simulink model "mamapwm"  (R2013a)
settings: Solver=ode45  StartTime=0.0  StopTime=1.4  RelTol=1e-3
libraries: simulink x1
settings Model: Creator=leGaly  LastModifiedBy=leGaly

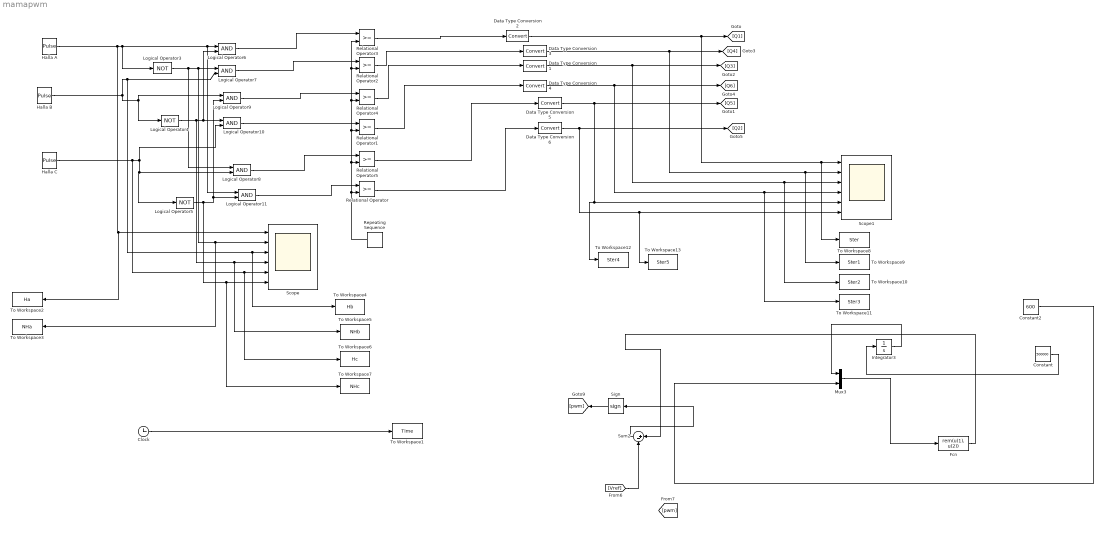
== system mamapwm ==
  Clock : Clock
  Constant : Constant  Value=500000
  Constant2 : Constant  Value=600
  Data Type Conversion{1..6} (6 alike) : DataTypeConversion
  Fcn : Fcn  Expr=rem(u(1), u(2))
  Halla A : DiscretePulseGenerator  PulseType=Time based  Period=0.6  PulseWidth=50
  Halla B : DiscretePulseGenerator  PulseType=Time based  Period=0.6  PulseWidth=50  PhaseDelay=0.2
  Halla C : DiscretePulseGenerator  PulseType=Time based  Period=0.6  PulseWidth=50  PhaseDelay=-0.2
  Integrator3 : Integrator
  Logical Operator{6..11} (6 alike) : Logic  AllPortsSameDT=off  OutDataTypeStr=boolean
  Logical Operator3 : Logic  Operator=NOT  AllPortsSameDT=off  OutDataTypeStr=boolean
  Logical Operator4 : Logic  Operator=NOT  AllPortsSameDT=off  OutDataTypeStr=boolean
  Logical Operator5 : Logic  Operator=NOT  AllPortsSameDT=off  OutDataTypeStr=boolean
  Mux3 : Mux  Inputs=2
  Relational Operator{,1..5} (6 alike) : RelationalOperator  OutDataTypeStr=boolean
  Repeating Sequence : simulink/Sources/Repeating Sequence  rep_seq_t=[0 12e-12]  rep_seq_y=[0.0001 1.5]
  Scope : Scope  NumInputPorts=6
      settings: YMin=-5~-5~-5~-5~-5~-5  YMax=5~5~5~5~5~5
  Scope1 : Scope  NumInputPorts=6
      settings: YMin=-5~-5~-5~-5~-5~-5  YMax=5~5~5~5~5~5
  Sign : Signum
  Sum2 : Sum  Inputs=|+-
  To Workspace1 : ToWorkspace  VariableName=Time  SampleTime=-1  SaveFormat=Structure With Time
  To Workspace10 : ToWorkspace  VariableName=Ster2  SampleTime=-1  SaveFormat=Structure With Time
  To Workspace11 : ToWorkspace  VariableName=Ster3  SampleTime=-1  SaveFormat=Structure With Time
  To Workspace12 : ToWorkspace  VariableName=Ster4  SampleTime=-1  SaveFormat=Structure With Time
  To Workspace13 : ToWorkspace  VariableName=Ster5  SampleTime=-1  SaveFormat=Structure With Time
  To Workspace2 : ToWorkspace  VariableName=Ha  SampleTime=-1  SaveFormat=Structure With Time
  To Workspace3 : ToWorkspace  VariableName=NHa  SampleTime=-1  SaveFormat=Structure With Time
  To Workspace4 : ToWorkspace  VariableName=Hb  SampleTime=-1  SaveFormat=Structure With Time
  To Workspace5 : ToWorkspace  VariableName=NHb  SampleTime=-1  SaveFormat=Structure With Time
  To Workspace6 : ToWorkspace  VariableName=Hc  SampleTime=-1  SaveFormat=Structure With Time
  To Workspace7 : ToWorkspace  VariableName=NHc  SampleTime=-1  SaveFormat=Structure With Time
  To Workspace8 : ToWorkspace  VariableName=Ster  SampleTime=-1  SaveFormat=Structure With Time
  To Workspace9 : ToWorkspace  VariableName=Ster1  SampleTime=-1  SaveFormat=Structure With Time
  wires:
  Logical Operator4/1 -> To Workspace5/1, Scope/4, Logical Operator10/1, Logical Operator6/2
  Logical Operator3/1 -> To Workspace3/1, Scope/2, Logical Operator7/1, Logical Operator8/1
  Logical Operator5/1 -> To Workspace7/1, Scope/6, Logical Operator11/2, Logical Operator9/2
  Logical Operator6/1 -> Relational Operator3/1
  Logical Operator9/1 -> Relational Operator4/1
  Logical Operator10/1 -> Relational Operator1/1
  Logical Operator8/1 -> Relational Operator5/1
  Logical Operator11/1 -> Relational Operator/1
  Halla A/1 -> To Workspace2/1, Scope/1, Logical Operator3/1, Logical Operator11/1, Logical Operator6/1
  Halla B/1 -> To Workspace4/1, Scope/3, Logical Operator7/2, Logical Operator4/1, Logical Operator9/1
  Halla C/1 -> To Workspace6/1, Scope/5, Logical Operator5/1, Logical Operator8/2, Logical Operator10/2
  Constant/1 -> Integrator3/1
  Integrator3/1 -> Mux3/1
  Constant2/1 -> Mux3/2
  Mux3/1 -> Fcn/1
  Fcn/1 -> Sum2/1
  Sum2/1 -> Sign/1
  Sign/1 -> [pwm]
  [Vref] -> Sum2/2
  Data Type Conversion2/1 -> To Workspace8/1, Scope1/1, [Q1]
  Data Type Conversion3/1 -> To Workspace9/1, Scope1/2, [Q4]
  Data Type Conversion1/1 -> To Workspace10/1, Scope1/3, [Q3]
  Data Type Conversion4/1 -> To Workspace11/1, Scope1/4, [Q6]
  Data Type Conversion5/1 -> Scope1/5, To Workspace12/1, [Q5]
  Data Type Conversion6/1 -> To Workspace13/1, Scope1/6, [Q2]
  Clock/1 -> To Workspace1/1
  Logical Operator7/1 -> Relational Operator2/1
  Relational Operator2/1 -> Data Type Conversion3/1
  Relational Operator3/1 -> Data Type Conversion2/1
  Repeating Sequence/1 -> Relational Operator/2, Relational Operator5/2, Relational Operator1/2, Relational Operator4/2, Relational Operator2/2, Relational Operator3/2
  Relational Operator4/1 -> Data Type Conversion1/1
  Relational Operator1/1 -> Data Type Conversion4/1
  Relational Operator5/1 -> Data Type Conversion5/1
  Relational Operator/1 -> Data Type Conversion6/1
